simulink model "trenl"  (R2025b)
settings: Solver=VariableStepAuto  StartTime=0.0  StopTime=10.0  RelTol=1e-3
values from neighbouring files (symbols this model uses):
  Am = 201    [test.m]
  NP = fraceks(j,2)    [test.m]
  R = 42    [test.m]
  to = round(rand*100)    [test.m]
  Ts = 0.001    [test.m]
libraries: commanapbnd3 x2
settings Model: Creator=pavel  LastModifiedBy=pavel

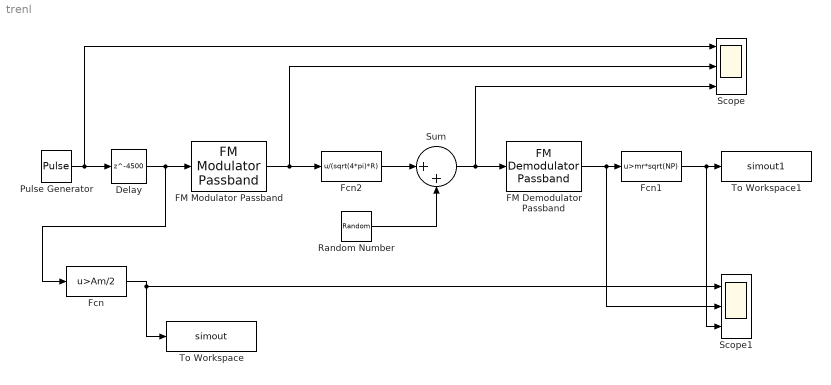
== system trenl ==
  Delay : Delay  DelayLength=4500  SampleTime=Ts
  FM Demodulator Passband : commanapbnd3/FM Demodulator Passband  Fc=fc  Ph=0  Kc=Am  Ho=100
  FM Modulator Passband : commanapbnd3/FM Modulator Passband  Fc=fc  Ph=0  Kc=Am
  Fcn : Fcn  Expr=u>Am/2
  Fcn1 : Fcn  Expr=u>mr*sqrt(NP)
  Fcn2 : Fcn  Expr=u/(sqrt(4*pi)*R)
  Pulse Generator : DiscretePulseGenerator  Amplitude=Am  Period=10  SampleTime=Ts
  Random Number : RandomNumber  Variance=NP  Seed=to  SampleTime=Ts
  Scope : Scope  NumInputPorts=3
      settings: ActiveDisplayYMinimum=-25.124999999999993  ActiveDisplayYMaximum=226.125
  Scope1 : Scope  NumInputPorts=3
      settings: ActiveDisplayYMinimum=-1  ActiveDisplayYMaximum=1
  Sum : Sum  Inputs=|++
  To Workspace : ToWorkspace  VariableName=simout  SampleTime=1
  To Workspace1 : ToWorkspace  VariableName=simout1  SampleTime=1
  wires:
  Pulse Generator/1 -> Scope/1, Delay/1
  Fcn2/1 -> Sum/1
  FM Modulator Passband/1 -> Scope/2, Fcn2/1
  Delay/1 -> FM Modulator Passband/1, Fcn/1
  Sum/1 -> FM Demodulator Passband/1, Scope/3
  FM Demodulator Passband/1 -> Scope1/2, Fcn1/1
  Fcn/1 -> To Workspace/1, Scope1/1
  Fcn1/1 -> Scope1/3, To Workspace1/1
  Random Number/1 -> Sum/2
